simulink model "ControladorP"  (R2023b)
settings: Solver=VariableStepAuto  StartTime=0.0  StopTime=10.0  RelTol=1e-3
settings Model: Creator=julia  LastModifiedBy=julia

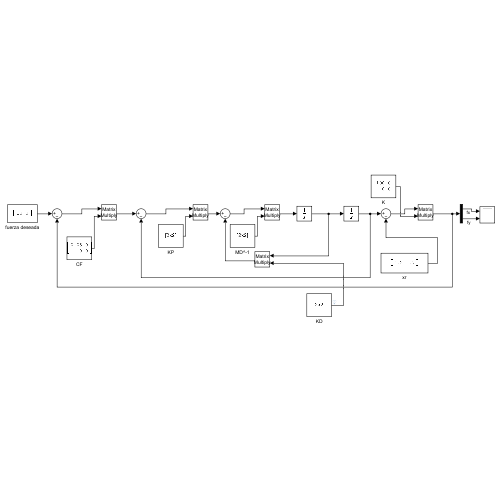
[thumbnail: Simulink's stored preview of the top-level diagram]
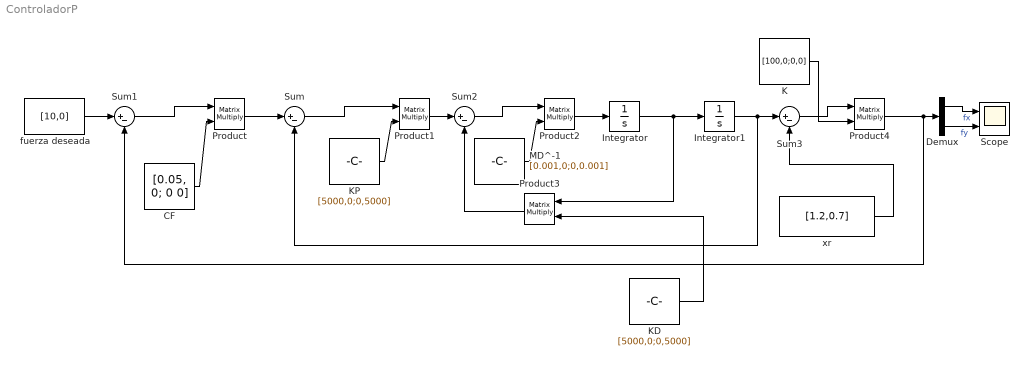
== system ControladorP ==
  CF : Constant  Value=[0.05, 0; 0 0]  VectorParams1D=off
  Demux : Demux  Outputs=2
  Integrator : Integrator  InitialCondition=[0,0]
  Integrator1 : Integrator  InitialCondition=[0,0]
  K : Constant  Value=[100,0;0,0]  VectorParams1D=off
  KD : Constant  Value=[5000,0;0,5000]  VectorParams1D=off
  KP : Constant  Value=[5000,0;0,5000]  VectorParams1D=off
  MD^-1 : Constant  Value=[0.001,0;0,0.001]  VectorParams1D=off
  Product{,1..4} (5 alike) : Product  Multiplication=Matrix(*)
  Scope : Scope  NumInputPorts=2
  Sum{,1..3} (4 alike) : Sum  Inputs=|+-
  fuerza deseada : Constant  Value=[10,0]  VectorParams1D=off
  xr : Constant  Value=[1.2,0.7]  VectorParams1D=off
  wires:
  Product4/1 -> Demux/1, Sum1/2
  Sum1/1 -> Product/1
  Product1/1 -> Sum2/1
  Sum3/1 -> Product4/1
  Product/1 -> Sum/1
  KP/1 -> Product1/2
  KD/1 -> Product3/2
  Demux/1 -> Scope/1  "fx"
  Sum2/1 -> Product2/1
  Product2/1 -> Integrator/1
  MD^-1/1 -> Product2/2
  Sum/1 -> Product1/1
  Demux/2 -> Scope/2  "fy"
  K/1 -> Product4/2
  Integrator/1 -> Product3/1, Integrator1/1
  xr/1 -> Sum3/2
  fuerza deseada/1 -> Sum1/1
  Product3/1 -> Sum2/2
  Integrator1/1 -> Sum3/1, Sum/2
  CF/1 -> Product/2
